simulink model "globe_simulator"  (R2022a)
settings: Solver=VariableStepAuto  StartTime=0.0  StopTime=tmax  MaxStep=dt  RelTol=1e-3
values from neighbouring files (symbols this model uses):
  inclination = 80*rad    (= 1.3962634016)    [globe_test.m]    (also in main.m = 0.174532925199)
  r0 = r_earth+launch_altitude    [globe_test.m]
  r_earth = 6.3781*10^6    (= 6378100)    [planet.m]
  theta0 = 0*rad    (= 0)    [globe_test.m]
  V0 = 8200    [globe_test.m]
undefined symbols (not defined in the file or in its folder): gm
libraries: simulink x1
settings Model: Creator=mitch  LastModifiedBy=mitch
settings DataIOCC: ReturnWorkspaceOutputs=off

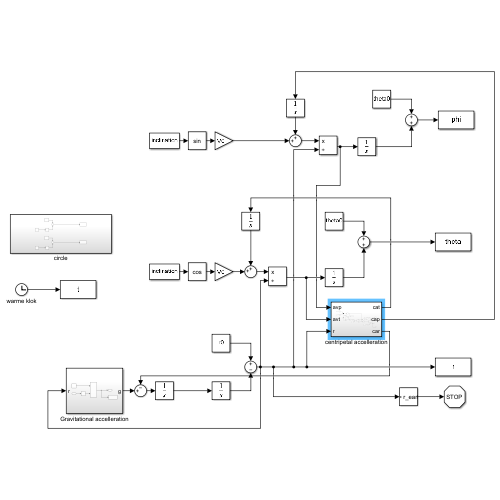
[thumbnail: Simulink's stored preview of the top-level diagram]
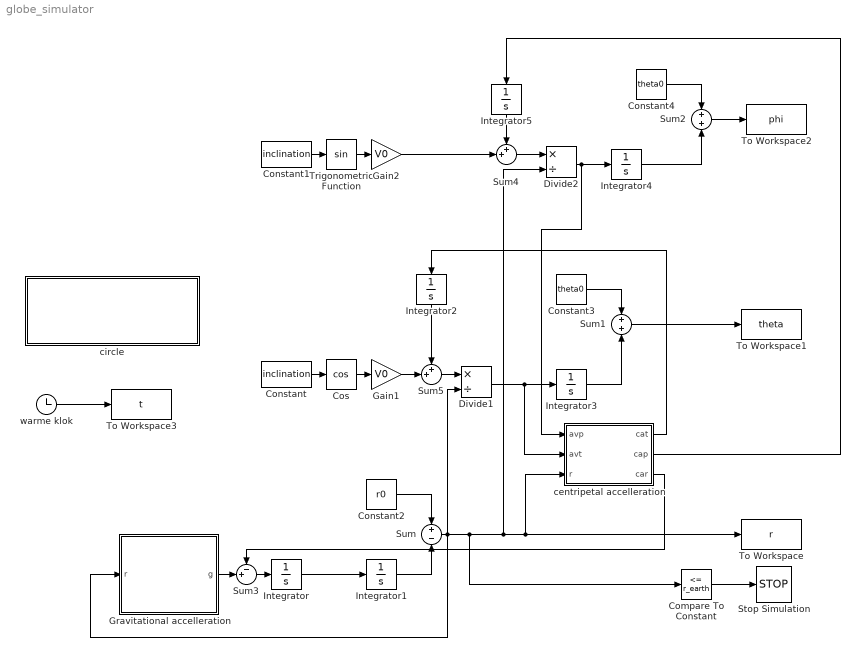
== system globe_simulator ==
  Compare To Constant : simulink/Logic and Bit Operations/Compare To Constant  relop=<=  const=r_earth  OutDataTypeStr=boolean
  Constant : Constant  Value=inclination
  Constant1 : Constant  Value=inclination
  Constant2 : Constant  Value=r0
  Constant3 : Constant  Value=theta0
  Constant4 : Constant  Value=theta0
  Cos : Trigonometry  Operator=cos
  Divide1 : Product  Inputs=*/
  Divide2 : Product  Inputs=*/
  Gain1 : Gain  Gain=V0
  Gain2 : Gain  Gain=V0
  Gravitational accelleration : Subsystem
  Integrator{,1..5} (6 alike) : Integrator
  Stop Simulation : Stop
  Sum : Sum  Inputs=+-
  Sum1 : Sum
  Sum2 : Sum
  Sum3 : Sum  Inputs=-+|
  Sum4 : Sum  Inputs=++|
  Sum5 : Sum  Inputs=++|
  To Workspace : ToWorkspace  VariableName=r  SampleTime=-1
  To Workspace1 : ToWorkspace  VariableName=theta  SampleTime=-1
  To Workspace2 : ToWorkspace  VariableName=phi  SampleTime=-1
  To Workspace3 : ToWorkspace  VariableName=t  SampleTime=-1
  Trigonometric Function : Trigonometry
  centripetal accelleration : Subsystem
  circle : Subsystem
  warme klok : Clock
  wires:
  Integrator/1 -> Integrator1/1
  Sum/1 -> Divide1/2, Gravitational accelleration/1(r), Compare To Constant/1, To Workspace/1, centripetal accelleration/3(r), Divide2/2
  Constant2/1 -> Sum/1
  Integrator1/1 -> Sum/2
  Sum1/1 -> To Workspace1/1
  Constant3/1 -> Sum1/1
  Integrator3/1 -> Sum1/2
  Compare To Constant/1 -> Stop Simulation/1
  warme klok/1 -> To Workspace3/1
  Sum3/1 -> Integrator/1
  Gravitational accelleration/1(g) -> Sum3/2
  centripetal accelleration/3(car) -> Sum3/1
  Divide1/1 -> Integrator3/1, centripetal accelleration/2(avt)
  centripetal accelleration/1(cat) -> Integrator2/1
  Sum5/1 -> Divide1/1
  Gain1/1 -> Sum5/2
  Constant/1 -> Cos/1
  Cos/1 -> Gain1/1
  Constant1/1 -> Trigonometric Function/1
  Trigonometric Function/1 -> Gain2/1
  Gain2/1 -> Sum4/2
  Sum4/1 -> Divide2/1
  Divide2/1 -> Integrator4/1, centripetal accelleration/1(avp)
  Constant4/1 -> Sum2/1
  Integrator4/1 -> Sum2/2
  Sum2/1 -> To Workspace2/1
  centripetal accelleration/2(cap) -> Integrator5/1
  Integrator5/1 -> Sum4/1
  Integrator2/1 -> Sum5/1

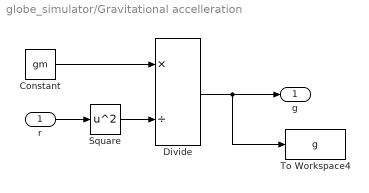
== system globe_simulator/Gravitational accelleration ==
  r : Inport
  Constant : Constant  Value=gm
  Divide : Product  Inputs=*/
  Square : Math  Operator=square
  To Workspace4 : ToWorkspace  VariableName=g  SampleTime=-1
  g : Outport
  wires:
  Divide/1 -> g/1, To Workspace4/1
  Square/1 -> Divide/2
  Constant/1 -> Divide/1
  r/1 -> Square/1

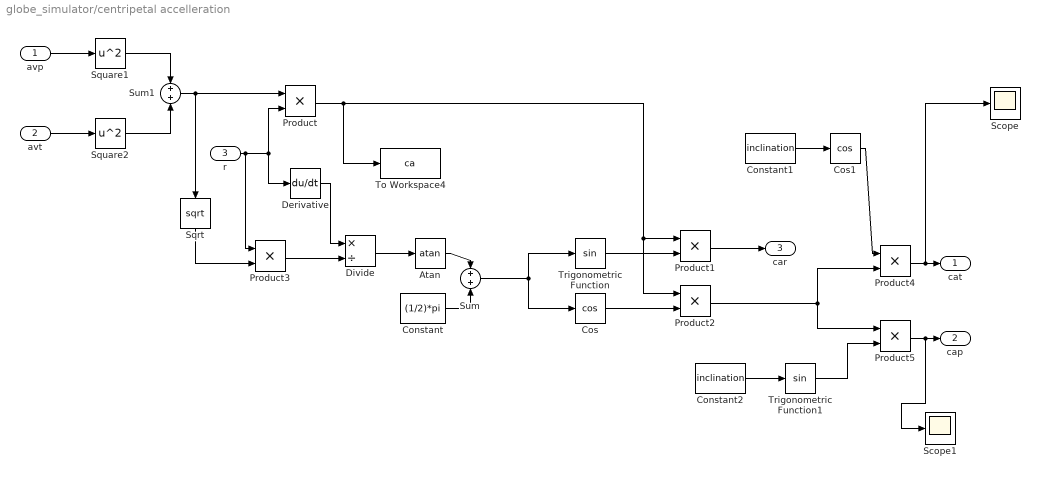
== system globe_simulator/centripetal accelleration ==
  avp : Inport
  avt : Inport  Port=2
  r : Inport  Port=3
  Atan : Trigonometry  Operator=atan
  Constant : Constant  Value=(1/2)*pi
  Constant1 : Constant  Value=inclination
  Constant2 : Constant  Value=inclination
  Cos : Trigonometry  Operator=cos
  Cos1 : Trigonometry  Operator=cos
  Derivative : Derivative
  Divide : Product  Inputs=*/
  Product{,1..5} (6 alike) : Product
  Scope : Scope
  Scope1 : Scope
  Sqrt : Sqrt
  Square1 : Math  Operator=square
  Square2 : Math  Operator=square
  Sum : Sum
  Sum1 : Sum
  To Workspace4 : ToWorkspace  VariableName=ca  SampleTime=-1
  Trigonometric Function : Trigonometry
  Trigonometric Function1 : Trigonometry
  cat : Outport
  cap : Outport  Port=2
  car : Outport  Port=3
  wires:
  Sum1/1 -> Sqrt/1, Product/1
  r/1 -> Product3/1, Derivative/1, Product/2
  Product/1 -> To Workspace4/1, Product2/1, Product1/1
  Divide/1 -> Atan/1
  Constant/1 -> Sum/2
  Atan/1 -> Sum/1
  Sum/1 -> Cos/1, Trigonometric Function/1
  Trigonometric Function/1 -> Product1/2
  Cos/1 -> Product2/2
  Product1/1 -> car/1
  Derivative/1 -> Divide/1
  Product3/1 -> Divide/2
  avp/1 -> Square1/1
  avt/1 -> Square2/1
  Square1/1 -> Sum1/1
  Square2/1 -> Sum1/2
  Sqrt/1 -> Product3/2
  Constant2/1 -> Trigonometric Function1/1
  Trigonometric Function1/1 -> Product5/2
  Product2/1 -> Product5/1, Product4/2
  Product5/1 -> Scope1/1, cap/1
  Product4/1 -> Scope/1, cat/1
  Constant1/1 -> Cos1/1
  Cos1/1 -> Product4/1

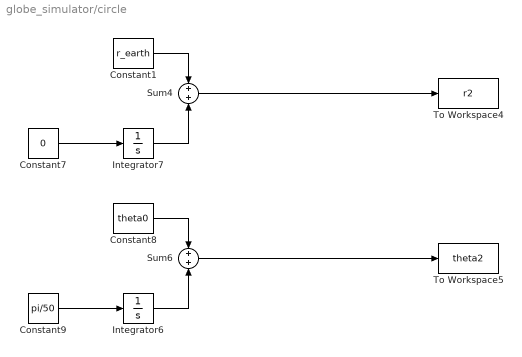
== system globe_simulator/circle ==
  Constant1 : Constant  Value=r_earth
  Constant7 : Constant  Value=0
  Constant8 : Constant  Value=theta0
  Constant9 : Constant  Value=pi/50
  Integrator6 : Integrator
  Integrator7 : Integrator
  Sum4 : Sum
  Sum6 : Sum
  To Workspace4 : ToWorkspace  VariableName=r2  SampleTime=-1
  To Workspace5 : ToWorkspace  VariableName=theta2  SampleTime=-1
  wires:
  Constant7/1 -> Integrator7/1
  Integrator7/1 -> Sum4/2
  Constant9/1 -> Integrator6/1
  Sum4/1 -> To Workspace4/1
  Constant8/1 -> Sum6/1
  Integrator6/1 -> Sum6/2
  Constant1/1 -> Sum4/1
  Sum6/1 -> To Workspace5/1
